simulink model "MAS240Hysterese"  (R2023b)
settings: Solver=FixedStepAuto  StartTime=0.0  StopTime=inf  RelTol=1e-3  EnableMultiTasking=on
model workspace (MAT data in the model file):
  hysterese = 2.5
libraries: arduinolib x2
settings Model: ExtModeTrigDuration=2  Creator=haava  LastModifiedBy=haava
settings OptimizationCC: EnhancedBackFolding=on  PassReuseOutputArgsAs=Individual arguments  ZeroExternalMemoryAtStartup=off  ZeroInternalMemoryAtStartup=off  MaxStackSize=64  OptimizeBlockOrder=speed  DifferentSizesBufferReuse=on  OptimizationCustomize=off  EfficientTunableParamExpr=on
settings DebuggingCC: ParameterTunabilityLossMsg=error
settings HardwareCC: ProdBitPerInt=16  ProdBitPerPointer=16  ProdBitPerSizeT=16  ProdBitPerPtrDiffT=16  ProdLargestAtomicFloat=None  ProdWordSize=8  ProdHWDeviceType=Atmel->AVR  UseEmbeddedCoderFeatures=off  UseSimulinkCoderFeatures=off
settings SFSimCC: MATLABDynamicMemAlloc=off
settings RTWCC: Description=Embedded Coder  SystemTargetFile=ert.tlc  HardwareBoard=Arduino Mega 2560  TemplateMakefile=ert_default_tmf  Toolchain=Arduino AVR  BuildConfiguration=Faster Runs
settings CodeAppCC: ForceParamTrailComments=on  IgnoreCustomStorageClasses=off  OperatorAnnotations=on  SimulinkDataObjDesc=on  SFDataObjDesc=on  InsertBlockDesc=on
settings ERTTargetCC: SupportContinuousTime=on  SupportNonInlinedSFcns=on  SupportVariableSizeSignals=on  ExtModeTransport=3  ExtModeStaticAlloc=on  ExtModeAutomaticAllocSize=off  ExtModeStaticAllocSize=2048  ExtModeMexFile=ext_xcp  ExtModeIntrfLevel=Level2 - Open

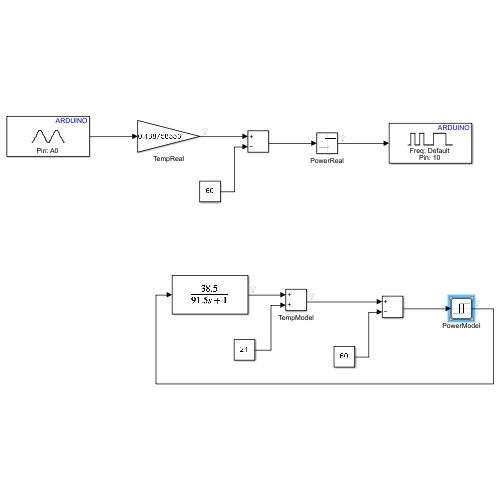
[thumbnail: Simulink's stored preview of the top-level diagram]
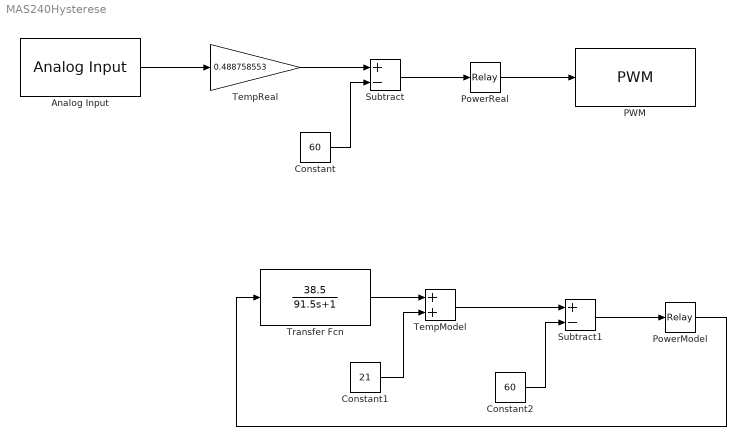
== system MAS240Hysterese ==
  Analog Input : arduinolib/Analog Input  pinNumber=0  ReadResultsOnly=off  ConversionTriggerSource=Software  ExternalTriggerType=uint32( 0 )  OutputDataType=uint16  EnableConversionCompleteNotify=off  EnableOuputStatus=off  SampleTime=-1  blockPlatform=arduino
  Constant : Constant  Value=60
  Constant1 : Constant  Value=21
  Constant2 : Constant  Value=60
  PWM : arduinolib/PWM  pinNumber=10  frequencyType=Default  desiredFrequency=490.2  achievableFrequency=490.2
  PowerModel : Relay  OnSwitchValue=2.5  OffSwitchValue=-2.5  OnOutputValue=0  OffOutputValue=3.794
  PowerReal : Relay  OnSwitchValue=2.5  OffSwitchValue=-2.5  OnOutputValue=0  OffOutputValue=255
  Subtract : Sum  Inputs=+-
  Subtract1 : Sum  Inputs=+-
  TempModel : Sum
  TempReal : Gain  Gain=0.488758553
  Transfer Fcn : TransferFcn  Numerator=[38.5]  Denominator=[91.5 1]
  wires:
  Analog Input/1 -> TempReal/1
  TempReal/1 -> Subtract/1
  Subtract/1 -> PowerReal/1
  Constant/1 -> Subtract/2
  PowerReal/1 -> PWM/1
  Transfer Fcn/1 -> TempModel/1
  Constant1/1 -> TempModel/2
  Constant2/1 -> Subtract1/2
  Subtract1/1 -> PowerModel/1
  TempModel/1 -> Subtract1/1
  PowerModel/1 -> Transfer Fcn/1
